simulink model "double_pendulum"  (R2024b)
settings: Solver=ode45  StartTime=0.0  StopTime=15.0  MaxStep=2^-5  RelTol=1e-3
settings Model: Creator=zv53855  LastModifiedBy=zv53855

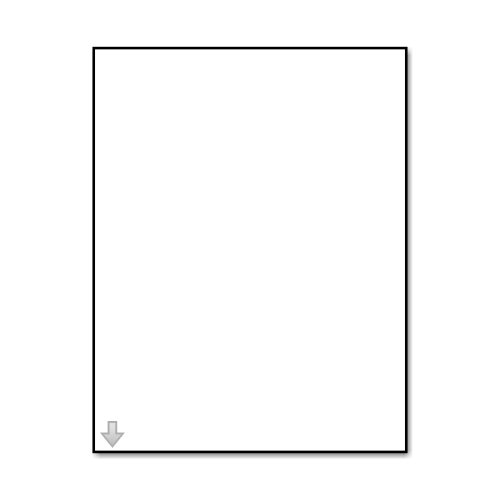
[thumbnail: Simulink's stored preview of the top-level diagram]
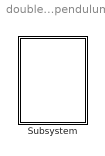
== system double_pendulum ==
  Subsystem : Subsystem  mask{g=9.81, k1=2, k2=1, m1=1, m2=2, l1=1, l2=2, phi1_1=80*pi/180, phi1_2=0*pi/180, phi2_1=150*pi/180, phi2_2=0*pi/180}
      mask prompts: k1 "k_1"; k2 "k_2"; m1 "mass 1"; m2 "mass 2"; l1 "rod 1"; l2 "rod 2"; phi1_1 "pendulum 1 speed"; phi1_2 "pendulum 1 acceleration"; phi2_1 "pendulum 2 speed"; phi2_2 "pendulum 2 acceleration"

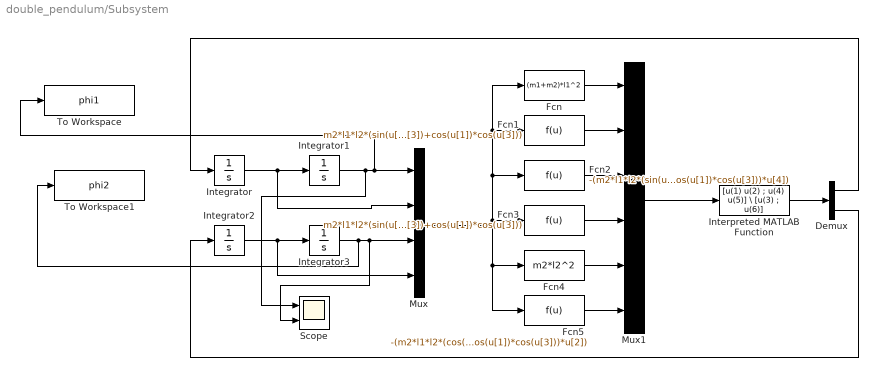
== system double_pendulum/Subsystem ==
  Demux : Demux  Outputs=2
  Fcn : Fcn  Expr=(m1+m2)*l1^2
  Fcn1 : Fcn  Expr=m2*l1*l2*(sin(u[1])*sin(u[3])+cos(u[1])*cos(u[3]))
  Fcn2 : Fcn  Expr=-(m2*l1*l2*(sin(u[1])*cos(u[3])-cos(u[1])*sin(u[3]))*u[4]^2 + (m1+m2)*g*l1*sin(u[1]) + k1*l1^2*u[2] + k2*l1*l2*(sin(u[1])*sin(u[3])+cos(u[1])*cos(u[3]))*u[4])
  Fcn3 : Fcn  Expr=m2*l1*l2*(sin(u[1])*sin(u[3])+cos(u[1])*cos(u[3]))
  Fcn4 : Fcn  Expr=m2*l2^2
  Fcn5 : Fcn  Expr=-(m2*l1*l2*(cos(u[1])*sin(u[3])-sin(u[1])*cos(u[3]))*u[2]^2 + m2*g*l2*sin(u[3]) + k2*l2^2*u[4] + k2*l1*l2*(sin(u[1])*sin(u[3])+cos(u[1])*cos(u[3]))*u[2])
  Integrator : Integrator  InitialCondition=phi1_2
  Integrator1 : Integrator  InitialCondition=phi1_1
  Integrator2 : Integrator  InitialCondition=phi2_2
  Integrator3 : Integrator  InitialCondition=phi2_1
  Interpreted MATLAB Function : MATLABFcn  MATLABFcn=[u(1) u(2) ; u(4) u(5)] \ [u(3) ; u(6)]
  Mux : Mux
  Mux1 : Mux  Inputs=6
  Scope : Scope  NumInputPorts=2
  To Workspace : ToWorkspace  VariableName=phi1  SampleTime=-1
  To Workspace1 : ToWorkspace  VariableName=phi2  SampleTime=-1
  wires:
  Integrator1/1 -> Scope/1, To Workspace/1, Mux/1
  Integrator2/1 -> Integrator3/1, Mux/4
  Integrator/1 -> Integrator1/1, Mux/2
  Mux/1 -> Fcn/1, Fcn1/1, Fcn2/1, Fcn3/1, Fcn5/1, Fcn4/1
  Fcn5/1 -> Mux1/6
  Fcn4/1 -> Mux1/5
  Fcn3/1 -> Mux1/4
  Fcn2/1 -> Mux1/3
  Fcn1/1 -> Mux1/2
  Fcn/1 -> Mux1/1
  Mux1/1 -> Interpreted MATLAB Function/1
  Interpreted MATLAB Function/1 -> Demux/1
  Demux/1 -> Integrator/1
  Demux/2 -> Integrator2/1
  Integrator3/1 -> To Workspace1/1, Scope/2, Mux/3
